simulink model "SF009A_DutyCycThermProtn"  (R2013b)
settings: Solver=FixedStepDiscrete  SolverMode=SingleTasking  StartTime=0.0  StopTime=1  FixedStep=0.1  RelTol=1e-3
values from neighbouring files (symbols this model uses):
  AbsltTThermLimCnt = DataDict.NTC    [SF009A_DutyCycThermProtn_DataDict.m]
  ARCHGLBPRM_100MILLISEC_SEC_F32 = DataDict.Constant    [SF009A_DutyCycThermProtn_DataDict.m]
  CTRLRANDCUTFLT_CNT_U08 = DataDict.Constant    [SF009A_DutyCycThermProtn_DataDict.m]
  CTRLRTFLT_CNT_U08 = DataDict.Constant    [SF009A_DutyCycThermProtn_DataDict.m]
  CUTFLT_CNT_U08 = DataDict.Constant    [SF009A_DutyCycThermProtn_DataDict.m]
  DITHERMLIM_MOTNWTMTR_F32 = DataDict.Constant    [SF009A_DutyCycThermProtn_DataDict.m]
  DutyCycExcddCnt = DataDict.NTC    [SF009A_DutyCycThermProtn_DataDict.m]
  DutyCycThermProtnAbsltCtrlTTblX = DataDict.Calibration    [SF009A_DutyCycThermProtn_DataDict.m]
  DutyCycThermProtnAbsltCtrlTTqTblY = DataDict.Calibration    [SF009A_DutyCycThermProtn_DataDict.m]
  DutyCycThermProtnAbsltCuTTblX = DataDict.Calibration    [SF009A_DutyCycThermProtn_DataDict.m]
  DutyCycThermProtnAbsltCuTTqTblY = DataDict.Calibration    [SF009A_DutyCycThermProtn_DataDict.m]
  DutyCycThermProtnAbsltMotVelBreakPt = DataDict.Calibration    [SF009A_DutyCycThermProtn_DataDict.m]
  DutyCycThermProtnAbsltTTqSlewHiLim = DataDict.Calibration    [SF009A_DutyCycThermProtn_DataDict.m]
  DutyCycThermProtnAbsltTTqSlewLoLim = DataDict.Calibration    [SF009A_DutyCycThermProtn_DataDict.m]
  DutyCycThermProtnCtrlT = DataDict.Calibration    [SF009A_DutyCycThermProtn_DataDict.m]
  DutyCycThermProtnCtrlTSeln = DataDict.Calibration    [SF009A_DutyCycThermProtn_DataDict.m]
  DutyCycThermProtnDutyCycFildThd = DataDict.Calibration    [SF009A_DutyCycThermProtn_DataDict.m]
  DutyCycThermProtnIgnOffCtrlEna = DataDict.Calibration    [SF009A_DutyCycThermProtn_DataDict.m]
  DutyCycThermProtnIgnOffMsgWaitTi = DataDict.Calibration    [SF009A_DutyCycThermProtn_DataDict.m]
  DutyCycThermProtnLstTblValNonStall = DataDict.Calibration    [SF009A_DutyCycThermProtn_DataDict.m]
  DutyCycThermProtnLstTblValStall = DataDict.Calibration    [SF009A_DutyCycThermProtn_DataDict.m]
  DutyCycThermProtnMotPrTSeln = DataDict.Calibration    [SF009A_DutyCycThermProtn_DataDict.m]
  DutyCycThermProtnMplr1NonStallTblY = DataDict.Calibration    [SF009A_DutyCycThermProtn_DataDict.m]
  DutyCycThermProtnMplr1StallTblY = DataDict.Calibration    [SF009A_DutyCycThermProtn_DataDict.m]
  DutyCycThermProtnMplr2NonStallTblY = DataDict.Calibration    [SF009A_DutyCycThermProtn_DataDict.m]
  DutyCycThermProtnMplr2StallTblY = DataDict.Calibration    [SF009A_DutyCycThermProtn_DataDict.m]
  DutyCycThermProtnMplr3NonStallTblY = DataDict.Calibration    [SF009A_DutyCycThermProtn_DataDict.m]
  DutyCycThermProtnMplr3StallTblY = DataDict.Calibration    [SF009A_DutyCycThermProtn_DataDict.m]
  DutyCycThermProtnMplr4NonStallTblY = DataDict.Calibration    [SF009A_DutyCycThermProtn_DataDict.m]
  DutyCycThermProtnMplr4StallTblY = DataDict.Calibration    [SF009A_DutyCycThermProtn_DataDict.m]
  DutyCycThermProtnMplr5NonStallTblY = DataDict.Calibration    [SF009A_DutyCycThermProtn_DataDict.m]
  DutyCycThermProtnMplr5StallTblY = DataDict.Calibration    [SF009A_DutyCycThermProtn_DataDict.m]
  DutyCycThermProtnMplr6NonStallTblY = DataDict.Calibration    [SF009A_DutyCycThermProtn_DataDict.m]
  DutyCycThermProtnMplr6StallTblY = DataDict.Calibration    [SF009A_DutyCycThermProtn_DataDict.m]
  DutyCycThermProtnMplrTblX = DataDict.Calibration    [SF009A_DutyCycThermProtn_DataDict.m]
  DutyCycThermProtnMplrTSeln = DataDict.Calibration    [SF009A_DutyCycThermProtn_DataDict.m]
  DutyCycThermProtnSlowFilTSeln = DataDict.Calibration    [SF009A_DutyCycThermProtn_DataDict.m]
  DutyCycThermProtnThermLimScaFac = DataDict.Calibration    [SF009A_DutyCycThermProtn_DataDict.m]
  DutyCycThermProtnThermLoadLimTblX = DataDict.Calibration    [SF009A_DutyCycThermProtn_DataDict.m]
  DutyCycThermProtnThermLoadLimTblY = DataDict.Calibration    [SF009A_DutyCycThermProtn_DataDict.m]
  DutyCycThermProtnTqCmdSlewDwn = DataDict.Calibration    [SF009A_DutyCycThermProtn_DataDict.m]
  DutyCycThermProtnTqCmdSlewUp = DataDict.Calibration    [SF009A_DutyCycThermProtn_DataDict.m]
  FILVALMIN_ULS_F32 = DataDict.Constant    [SF009A_DutyCycThermProtn_DataDict.m]
  IGNTIOFFTHD_CNT_F32 = DataDict.Constant    [SF009A_DutyCycThermProtn_DataDict.m]
  NODEBSTEP_CNT_U16 = DataDict.Constant    [SF009A_DutyCycThermProtn_DataDict.m]
  ONEPERC_ULS_F32 = DataDict.Constant    [SF009A_DutyCycThermProtn_DataDict.m]
  TAU3_SEC_F32 = DataDict.Constant    [SF009A_DutyCycThermProtn_DataDict.m]
  TAU4_SEC_F32 = DataDict.Constant    [SF009A_DutyCycThermProtn_DataDict.m]
  TAU5_SEC_F32 = DataDict.Constant    [SF009A_DutyCycThermProtn_DataDict.m]
  TAU6_SEC_F32 = DataDict.Constant    [SF009A_DutyCycThermProtn_DataDict.m]
  THERMLOADLIMTBLIDX_ULS_U08 = DataDict.Constant    [SF009A_DutyCycThermProtn_DataDict.m]
undefined symbols (not defined in the file or in its folder): NtcSts1, NvmGetErrSts1
libraries: FixdToFloat x13, Fil x12, NxtrLim x12, simulink x11, NxtrMath x8, FloatToFixd x6, NxtrMax x6, NxtrMin x3, NxtrAbslt x2, NxtrNvM x1
(part 3 of 7)

== system SF009A_DutyCycThermProtn/DutyCycThermProtn/DutyCycThermProtnPer1/ThermalLimitStatus ==
  DutyCycThermProtnDi : Inport
  ThermLim : Inport  Port=2
  Maxout : Inport  Port=3
  CopyRight2 : Subsystem  Description=|  mask(Copyright Information){none=on}
      | Copyright info block.                                               
      |                                                                     
      | Place copyright information at the top of every subsystem in design.
      mask prompts: none "No parameters"
      mask help: Place copyright information at the top of every subsystem in design.
      mask Display:
      | NxtrConf = 'Nexteer Confidential';
      | 
      | sys = bdroot; %handle for the current model ("system")
      | first = get_param(sys,'Created');
      | if(isempty(first))
      |     first = datestr(now,'yyyy');
      | else
      |     first = first(end-3:end);  %year is last four digits
      | end
      | 
      | last = get_param(sys,'LastModifiedDate');
      | if isempty(last)
      |     last = datestr(now,'yyyy');
      | else
      |     last = last(end-3:end);
      | end
      | 
      | if strcmp(first,last)
      |     fprintf('%s -- Copyright %s Nexteer',NxtrConf,first)
      | else
      |     fprintf('%s -- %s%s- %s Nexteer',NxtrConf,char(169),first,last)
      | end
  DutyCycThermProtnDisabled : Subsystem  RequirementInfo={'linktype_rmi_doors' '0000a52a (/E-STEER Core/SubSystem Specifications/Application Functions/SF009A Thermal Duty Cycle Protection)' '#SF009A_267' 'true' 'REQ: SF009A_267' '' } %GIDa_3170260b_8ef3_42fb_9ac5_2884277200d1  TreatAsAtomicUnit=on
  "DutyCycThermProtnEnabled " : Subsystem  RequirementInfo={'linktype_rmi_doors' '0000a52a (/E-STEER Core/SubSystem Specifications/Application Functions/SF009A Thermal Duty Cycle Protection)' '#SF009A_235' 'true' 'REQ: SF009A_235' '' } %GIDa_8d68070d_e413_42c4_a42a_5b349cac34de  TreatAsAtomicUnit=on
  If2 : If  RequirementInfo={'linktype_rmi_doors' '0000a52a (/E-STEER Core/SubSystem Specifications/Application Functions/SF009A Thermal Duty Cycle Protection)' '#SF009A_267' 'true' 'REQ: SF009A_267' '' } %GIDa_d4c54a9c_c30e_44b1_8f16_11f79403e198  IfExpression=u1
  LimStat_f1 : NxtrLim/LimStat_f32  RequirementInfo={'linktype_rmi_doors' '0000a52a (/E-STEER Core/SubSystem Specifications/Application Functions/SF009A Thermal Duty Cycle Protection)' '#SF009A_205' 'true' 'REQ: SF009A_205' '' } %GIDa_2006209c_c7cf_49ec_9d42_30cb8989323e  LoLim=THERMREDNFACLOLIM_ULS_F32  HiLim=THERMREDNFACHILIM_ULS_F32
      settings: AttributesFormatString=Lower Limit: %<LoLim>\nUpper Limit: %<HiLim>
  MaxoutLimiting : Subsystem  RequirementInfo={'linktype_rmi_doors' '0000a52a (/E-STEER Core/SubSystem Specifications/Application Functions/SF009A Thermal Duty Cycle Protection)' '#SF009A_143' 'true' 'REQ: SF009A_143' '' } %GIDa_bba01dfd_191a_49a7_8d73_371fb59628a5  TreatAsAtomicUnit=on
  Merge2 : Merge  RequirementInfo={'linktype_rmi_doors' '0000a52a (/E-STEER Core/SubSystem Specifications/Application Functions/SF009A Thermal Duty Cycle Protection)' '#SF009A_267' 'true' 'REQ: SF009A_267' '' } %GIDa_1305f63a_c873_4a71_994b_19e3fb3df743
  ThermRednFac : Outport
  wires:
  DutyCycThermProtnDi/1 -> MaxoutLimiting/2(DutyCycThermProtnDi), If2/1
  DutyCycThermProtnDisabled/1(ThermRednFac) -> Merge2/1
  If2/1 -> DutyCycThermProtnDisabled/Action
  If2/2 -> "DutyCycThermProtnEnabled "/Action
  LimStat_f1/1 -> ThermRednFac/1
  Merge2/1 -> LimStat_f1/1
  "DutyCycThermProtnEnabled "/1(ThermRednFac) -> Merge2/2
  ThermLim/1 -> "DutyCycThermProtnEnabled "/1(ThermLim)
  Maxout/1 -> MaxoutLimiting/1(Maxout)

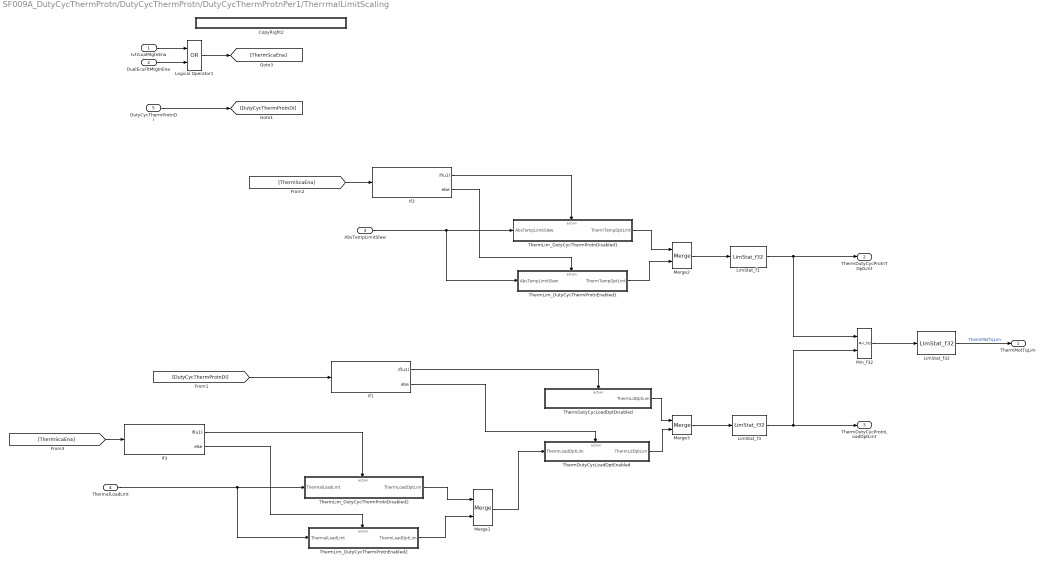
== system SF009A_DutyCycThermProtn/DutyCycThermProtn/DutyCycThermProtnPer1/TherrmalLimitScaling ==
  IvtrLoaMtgtnEna : Inport  RequirementInfo="{'linktype_rmi_doors' '0000a52a (/E-STEER Core/SubSystem Specifications/Application Functions/SF009A Thermal Duty Cycle Protection)' '#SF009A_312' 'true' 'REQ:  SF009A_312' '' } %GIDa_8dc61b0d_ff5c_4fa0_bf26_862789bc8c27"
  DualEcuFltMtgtnEna : Inport  RequirementInfo="{'linktype_rmi_doors' '0000a52a (/E-STEER Core/SubSystem Specifications/Application Functions/SF009A Thermal Duty Cycle Protection)' '#SF009A_312' 'true' 'REQ:  SF009A_312' '' } %GIDa_d897ebab_4d96_4080_9fe6_e7020e9fa09f"  Port=2
  AbsTempLimitSlew : Inport  Port=3
  ThermalLoadLmt : Inport  Port=4
  DutyCycThermProtnDi : Inport  Port=5
  CopyRight2 : Subsystem  Description=|  mask(Copyright Information){none=on}
      | Copyright info block.                                               
      |                                                                     
      | Place copyright information at the top of every subsystem in design.
      mask prompts: none "No parameters"
      mask help: Place copyright information at the top of every subsystem in design.
      mask Display:
      | NxtrConf = 'Nexteer Confidential';
      | 
      | sys = bdroot; %handle for the current model ("system")
      | first = get_param(sys,'Created');
      | first = first(end-3:end);  %year is last four digits
      | 
      | last = get_param(sys,'LastModifiedDate');
      | if isempty(last)
      |     last = datestr(now,'yyyy');
      | else
      |     last = last(end-3:end);
      | end
      | 
      | if strcmp(first,last)
      |     fprintf('%s -- Copyright %s Nexteer',NxtrConf,first)
      | else
      |     fprintf('%s -- %s%s- %s Nexteer',NxtrConf,char(169),first,last)
      | end
  If1 : If  RequirementInfo={} %GIDa_7babfb83_5b52_4390_b634_fda5df83494b  IfExpression=u1
  If2 : If  RequirementInfo={} %GIDa_2cee02fc_25df_4b08_940e_96d0c2f6e22c  IfExpression=u1
  If3 : If  RequirementInfo={} %GIDa_5f0eb570_64b4_4784_95d6_34c2b2a6baa7  IfExpression=u1
  LimStat_f1 : NxtrLim/LimStat_f32  RequirementInfo="{'linktype_rmi_doors' '0000a52a (/E-STEER Core/SubSystem Specifications/Application Functions/SF009A Thermal Duty Cycle Protection)' '#SF009A_309' 'true' 'REQ:  SF009A_309' '' } %GIDa_83c1db68_c9e1_4d9e_932e_8b8cb705e06f"  LoLim=ZERO_MOTNWTMTR_F32  HiLim=SYSGLBPRM_MOTTQCMDHILIM_MOTNWTMTR_F32
      settings: AttributesFormatString=Lower Limit: %<LoLim>\nUpper Limit: %<HiLim>
  LimStat_f3 : NxtrLim/LimStat_f32  RequirementInfo="{'linktype_rmi_doors' '0000a52a (/E-STEER Core/SubSystem Specifications/Application Functions/SF009A Thermal Duty Cycle Protection)' '#SF009A_317' 'true' 'REQ:  SF009A_317' '' } %GIDa_b846f976_f3d0_4532_b6c5_25ce29114272"  LoLim=ZERO_MOTNWTMTR_F32  HiLim=SYSGLBPRM_MOTTQCMDHILIM_MOTNWTMTR_F32
      settings: AttributesFormatString=Lower Limit: %<LoLim>\nUpper Limit: %<HiLim>
  LimStat_f32 : NxtrLim/LimStat_f32  RequirementInfo="{'linktype_rmi_doors' '0000a52a (/E-STEER Core/SubSystem Specifications/Application Functions/SF009A Thermal Duty Cycle Protection)' '#SF009A_318' 'true' 'REQ:  SF009A_318' '' ; 'linktype_rmi_doors' '0000a52a (/E-STEER Core/SubSystem Specifications/Application Functions/SF009A Thermal Duty Cycle Protection)' '#SF009A_319' 'true' 'REQ:  SF009A_319' '' } %GIDa_fa1de0a5_b024_4a72_90f6_53e74d27d671"  LoLim=ZERO_MOTNWTMTR_F32  HiLim=SYSGLBPRM_MOTTQCMDHILIM_MOTNWTMTR_F32
      settings: AttributesFormatString=Lower Limit: %<LoLim>\nUpper Limit: %<HiLim>
  Logical Operator1 : Logic  RequirementInfo="{'linktype_rmi_doors' '0000a52a (/E-STEER Core/SubSystem Specifications/Application Functions/SF009A Thermal Duty Cycle Protection)' '#SF009A_312' 'true' 'REQ:  SF009A_312' '' } %GIDa_a0ab542f_99be_4386_a7f5_35a00b0ad963"  Operator=OR  AllPortsSameDT=off  OutDataTypeStr=boolean
  Merge1 : Merge  RequirementInfo={} %GIDa_d5d1cf90_c902_44f9_82c6_0c36d1509e76
  Merge2 : Merge  RequirementInfo={} %GIDa_d9fd7fe5_0630_493a_b799_686d5074f1b6
  Merge3 : Merge  RequirementInfo={} %GIDa_28a261bc_f2e1_4059_b603_b96f360ef741
  Min_f32 : NxtrMin/Min_f32  SFunctionSpec=single y1 = Min_f32(single u1, single u2)
      settings: AttributesFormatString=%<Name>
  "ThermDutyCycLoadDptDisabled " : Subsystem  RequirementInfo="{'linktype_rmi_doors' '0000a52a (/E-STEER Core/SubSystem Specifications/Application Functions/SF009A Thermal Duty Cycle Protection)' '#SF009A_246' 'true' 'REQ:  SF009A_246' '' } %GIDa_ddc50ac8_1faa_42f8_93ea_c06be95ae3b1"  TreatAsAtomicUnit=on
  ThermDutyCycLoadDptEnabled : Subsystem  RequirementInfo="{'linktype_rmi_doors' '0000a52a (/E-STEER Core/SubSystem Specifications/Application Functions/SF009A Thermal Duty Cycle Protection)' '#SF009A_246' 'true' 'REQ:  SF009A_246' '' } %GIDa_c67cb7cb_e6e1_4854_8d46_a7dea79ca72f"  TreatAsAtomicUnit=on
  ThermLim_DutyCycThermProtnDisabled1 : Subsystem  RequirementInfo="{'linktype_rmi_doors' '0000a52a (/E-STEER Core/SubSystem Specifications/Application Functions/SF009A Thermal Duty Cycle Protection)' '#SF009A_313' 'true' 'REQ:  SF009A_313' '' } %GIDa_2586edea_1805_4e1d_ab84_f723d2ac45af"  TreatAsAtomicUnit=on
  ThermLim_DutyCycThermProtnDisabled2 : Subsystem  RequirementInfo="{'linktype_rmi_doors' '0000a52a (/E-STEER Core/SubSystem Specifications/Application Functions/SF009A Thermal Duty Cycle Protection)' '#SF009A_314' 'true' 'REQ:  SF009A_314' '' } %GIDa_45e1bc34_a818_4763_b74c_1022ecc67c55"  TreatAsAtomicUnit=on
  ThermLim_DutyCycThermProtnEnabled1 : Subsystem  RequirementInfo="{'linktype_rmi_doors' '0000a52a (/E-STEER Core/SubSystem Specifications/Application Functions/SF009A Thermal Duty Cycle Protection)' '#SF009A_313' 'true' 'REQ:  SF009A_313' '' } %GIDa_3bce7b55_05ff_4096_a1dc_b963e5e47b1a"  TreatAsAtomicUnit=on
  ThermLim_DutyCycThermProtnEnabled2 : Subsystem  RequirementInfo="{'linktype_rmi_doors' '0000a52a (/E-STEER Core/SubSystem Specifications/Application Functions/SF009A Thermal Duty Cycle Protection)' '#SF009A_314' 'true' 'REQ:  SF009A_314' '' } %GIDa_331a4316_f4e0_4847_8684_08c003b0afeb"  TreatAsAtomicUnit=on
  ThermMotTqLim : Outport  RequirementInfo="{'linktype_rmi_doors' '0000a52a (/E-STEER Core/SubSystem Specifications/Application Functions/SF009A Thermal Duty Cycle Protection)' '#SF009A_318' 'true' 'REQ:  SF009A_318' '' ; 'linktype_rmi_doors' '0000a52a (/E-STEER Core/SubSystem Specifications/Application Functions/SF009A Thermal Duty Cycle Protection)' '#SF009A_319' 'true' 'REQ:  SF009A_319' '' } %GIDa_a2d08e3e_eec7_4b12_a4b0_81f4b84f2415"
  ThermDutyCycProtnTDptLmt : Outport  RequirementInfo="{'linktype_rmi_doors' '0000a52a (/E-STEER Core/SubSystem Specifications/Application Functions/SF009A Thermal Duty Cycle Protection)' '#SF009A_309' 'true' 'REQ:  SF009A_309' '' } %GIDa_17b4566a_b19b_4e3d_9f2a_5a599306e544"  Port=2
  ThermDutyCycProtnLoadDptLmt : Outport  RequirementInfo="{'linktype_rmi_doors' '0000a52a (/E-STEER Core/SubSystem Specifications/Application Functions/SF009A Thermal Duty Cycle Protection)' '#SF009A_317' 'true' 'REQ:  SF009A_317' '' } %GIDa_b461d353_80d8_421a_910a_1fa039d560eb"  Port=3
  wires:
  LimStat_f32/1 -> ThermMotTqLim/1  "ThermMotTqLim"
  If1/1 -> "ThermDutyCycLoadDptDisabled "/Action
  If1/2 -> ThermDutyCycLoadDptEnabled/Action
  DutyCycThermProtnDi/1 -> [DutyCycThermProtnDi]
  "ThermDutyCycLoadDptDisabled "/1(ThermLdDptLim) -> Merge3/1
  ThermDutyCycLoadDptEnabled/1(ThermLdDptLim) -> Merge3/2
  Merge3/1 -> LimStat_f3/1
  LimStat_f3/1 -> Min_f32/2, ThermDutyCycProtnLoadDptLmt/1
  [DutyCycThermProtnDi] -> If1/1
  IvtrLoaMtgtnEna/1 -> Logical Operator1/1
  DualEcuFltMtgtnEna/1 -> Logical Operator1/2
  Logical Operator1/1 -> [ThermScaEna]
  [ThermScaEna] -> If2/1
  If2/1 -> ThermLim_DutyCycThermProtnDisabled1/Action
  AbsTempLimitSlew/1 -> ThermLim_DutyCycThermProtnEnabled1/1(AbsTempLimitSlew), ThermLim_DutyCycThermProtnDisabled1/1(AbsTempLimitSlew)
  If2/2 -> ThermLim_DutyCycThermProtnEnabled1/Action
  ThermLim_DutyCycThermProtnDisabled1/1(ThermTempDptLmt) -> Merge2/1
  ThermLim_DutyCycThermProtnEnabled1/1(ThermTempDptLmt) -> Merge2/2
  Merge2/1 -> LimStat_f1/1
  LimStat_f1/1 -> Min_f32/1, ThermDutyCycProtnTDptLmt/1
  [ThermScaEna] -> If3/1
  If3/1 -> ThermLim_DutyCycThermProtnDisabled2/Action
  ThermalLoadLmt/1 -> ThermLim_DutyCycThermProtnEnabled2/1(ThermalLoadLmt), ThermLim_DutyCycThermProtnDisabled2/1(ThermalLoadLmt)
  If3/2 -> ThermLim_DutyCycThermProtnEnabled2/Action
  ThermLim_DutyCycThermProtnDisabled2/1(ThermLoadDptLim) -> Merge1/1
  ThermLim_DutyCycThermProtnEnabled2/1(ThermLoadDptLim) -> Merge1/2
  Merge1/1 -> ThermDutyCycLoadDptEnabled/1(ThermLoadDptLim)
  Min_f32/1 -> LimStat_f32/1

== system SF009A_DutyCycThermProtn/DutyCycThermProtn/DutyCycThermProtnInit1/FilStVal_SetRamBlockStatus/CopyRight2 ==

== system SF009A_DutyCycThermProtn/DutyCycThermProtn/DutyCycThermProtnInit1/NVM_NOK/CopyRight2 ==

== system SF009A_DutyCycThermProtn/DutyCycThermProtn/DutyCycThermProtnInit1/NVM_Ok/CopyRight2 ==

== system SF009A_DutyCycThermProtn/DutyCycThermProtn/DutyCycThermProtnInit1/PowerOnTasks/CopyRight2 ==

== system SF009A_DutyCycThermProtn/DutyCycThermProtn/DutyCycThermProtnInit1/PowerOnTasks/DefaultIgnOffTime ==
  Action Port : ActionPort  ActionType=else
  CopyRight2 : Subsystem  Description=|  mask(Copyright Information){none=on}
      | Copyright info block.                                               
      |                                                                     
      | Place copyright information at the top of every subsystem in design.
      mask prompts: none "No parameters"
      mask help: Place copyright information at the top of every subsystem in design.
      mask Display:
      | NxtrConf = 'Nexteer Confidential';
      | 
      | sys = bdroot; %handle for the current model ("system")
      | first = get_param(sys,'Created');
      | first = first(end-3:end);  %year is last four digits
      | 
      | last = get_param(sys,'LastModifiedDate');
      | if isempty(last)
      |     last = datestr(now,'yyyy');
      | else
      |     last = last(end-3:end);
      | end
      | 
      | if strcmp(first,last)
      |     fprintf('%s -- Copyright %s Nexteer',NxtrConf,first)
      | else
      |     fprintf('%s -- %s%s- %s Nexteer',NxtrConf,char(169),first,last)
      | end
  DefIgnOffTime1 : Constant  RequirementInfo={'linktype_rmi_doors' '0000a52a (/E-STEER Core/SubSystem Specifications/Application Functions/SF009A Thermal Duty Cycle Protection)' '#SF009A_285' 'true' 'REQ: SF009A_285' '' } %GIDa_1c1a8355_68c4_4a16_a698_2c7b860aa81f  Value=FILVALMIN_ULS_F32
  FiltSV3 : Outport  RequirementInfo={'linktype_rmi_doors' '0000a52a (/E-STEER Core/SubSystem Specifications/Application Functions/SF009A Thermal Duty Cycle Protection)' '#SF009A_285' 'true' 'REQ: SF009A_285' '' } %GIDa_f53f9a1c_8faf_4833_a80c_e2891c436a6f
  FiltSV4 : Outport  RequirementInfo={'linktype_rmi_doors' '0000a52a (/E-STEER Core/SubSystem Specifications/Application Functions/SF009A Thermal Duty Cycle Protection)' '#SF009A_285' 'true' 'REQ: SF009A_285' '' } %GIDa_7573da05_c607_444c_bff7_05b9be356769  Port=2
  FiltSV5 : Outport  RequirementInfo={'linktype_rmi_doors' '0000a52a (/E-STEER Core/SubSystem Specifications/Application Functions/SF009A Thermal Duty Cycle Protection)' '#SF009A_285' 'true' 'REQ: SF009A_285' '' } %GIDa_0a22d052_a9b5_4254_83f4_8f154e55c7ba  Port=3
  FiltSV6 : Outport  RequirementInfo={'linktype_rmi_doors' '0000a52a (/E-STEER Core/SubSystem Specifications/Application Functions/SF009A Thermal Duty Cycle Protection)' '#SF009A_285' 'true' 'REQ: SF009A_285' '' } %GIDa_7f0b1c6f_6523_47e0_8553_42c05ca6b0db  Port=4
  wires:
  DefIgnOffTime1/1 -> FiltSV3/1, FiltSV4/1, FiltSV6/1, FiltSV5/1

== system SF009A_DutyCycThermProtn/DutyCycThermProtn/DutyCycThermProtnInit1/PowerOnTasks/InputIgnOffTime ==
  note: RANGE CHECK, ENSURE VALUE IS BELOW A CONSTANT (10000)
  IgnTiOff : Inport
  Action Port : ActionPort  ActionType=then
  CopyRight2 : Subsystem  Description=|  mask(Copyright Information){none=on}
      | Copyright info block.                                               
      |                                                                     
      | Place copyright information at the top of every subsystem in design.
      mask prompts: none "No parameters"
      mask help: Place copyright information at the top of every subsystem in design.
      mask Display:
      | NxtrConf = 'Nexteer Confidential';
      | 
      | sys = bdroot; %handle for the current model ("system")
      | first = get_param(sys,'Created');
      | first = first(end-3:end);  %year is last four digits
      | 
      | last = get_param(sys,'LastModifiedDate');
      | if isempty(last)
      |     last = datestr(now,'yyyy');
      | else
      |     last = last(end-3:end);
      | end
      | 
      | if strcmp(first,last)
      |     fprintf('%s -- Copyright %s Nexteer',NxtrConf,first)
      | else
      |     fprintf('%s -- %s%s- %s Nexteer',NxtrConf,char(169),first,last)
      | end
  Data Store Read : DataStoreRead  DataStoreName=FilStVal  DataStoreElements=FilStVal.Fil3StVal
  Data Store Read1 : DataStoreRead  DataStoreName=FilStVal  DataStoreElements=FilStVal.Fil4StVal
  Data Store Read2 : DataStoreRead  DataStoreName=FilStVal  DataStoreElements=FilStVal.Fil5StVal
  Data Store Read3 : DataStoreRead  DataStoreName=FilStVal  DataStoreElements=FilStVal.Fil6StVal
  Filt3ExpDecay : Subsystem  RequirementInfo={} %GIDa_9f9f3f65_c145_44e4_82e5_fd713760ae68
  Filt4ExpDecay : Subsystem  RequirementInfo={} %GIDa_626963e8_8ecf_441f_b1c9_4240579d77f9
  Filt5ExpDecay : Subsystem  RequirementInfo={} %GIDa_9364c89b_18fa_4473_8499_21374c540da9
  Filt6ExpDecay : Subsystem  RequirementInfo={} %GIDa_8e6049b9_bd81_40a5_96f3_6037c184dcb3
  FiltSV3 : Outport
  FiltSV4 : Outport  Port=2
  FiltSV5 : Outport  Port=3
  FiltSV6 : Outport  Port=4
  wires:
  Filt3ExpDecay/1(FiltSV) -> FiltSV3/1
  Data Store Read/1 -> Filt3ExpDecay/2(FiltSVOrg)
  Filt4ExpDecay/1(FiltSV) -> FiltSV4/1
  Filt5ExpDecay/1(FiltSV) -> FiltSV5/1
  Data Store Read2/1 -> Filt5ExpDecay/2(FiltSVOrg)
  Filt6ExpDecay/1(FiltSV) -> FiltSV6/1
  Data Store Read3/1 -> Filt6ExpDecay/2(FiltSVOrg)
  Data Store Read1/1 -> Filt4ExpDecay/2(FiltSVOrg)
  IgnTiOff/1 -> Filt3ExpDecay/1(IgnTimeOffSel), Filt4ExpDecay/1(IgnTimeOffSel), Filt6ExpDecay/1(IgnTimeOffSel), Filt5ExpDecay/1(IgnTimeOffSel)

== system SF009A_DutyCycThermProtn/DutyCycThermProtn/DutyCycThermProtnInit1/SetInitialValueOfAbsTempLimitSlew/Copyright1 ==

== system SF009A_DutyCycThermProtn/DutyCycThermProtn/DutyCycThermProtnInit1/SetInitialValueOfLstTblValRateLimrStVari/Copyright1 ==

== system SF009A_DutyCycThermProtn/DutyCycThermProtn/DutyCycThermProtnPer1/FiltSVReinit/CopyRight2 ==

== system SF009A_DutyCycThermProtn/DutyCycThermProtn/DutyCycThermProtnPer1/FiltSVReinit/VehTiVldDisabled ==
  Action Port : ActionPort  ActionType=else
  CopyRight2 : Subsystem  Description=|  mask(Copyright Information){none=on}
      | Copyright info block.                                               
      |                                                                     
      | Place copyright information at the top of every subsystem in design.
      mask prompts: none "No parameters"
      mask help: Place copyright information at the top of every subsystem in design.
      mask Display:
      | NxtrConf = 'Nexteer Confidential';
      | 
      | sys = bdroot; %handle for the current model ("system")
      | first = get_param(sys,'Created');
      | first = first(end-3:end);  %year is last four digits
      | 
      | last = get_param(sys,'LastModifiedDate');
      | if isempty(last)
      |     last = datestr(now,'yyyy');
      | else
      |     last = last(end-3:end);
      | end
      | 
      | if strcmp(first,last)
      |     fprintf('%s -- Copyright %s Nexteer',NxtrConf,first)
      | else
      |     fprintf('%s -- %s%s- %s Nexteer',NxtrConf,char(169),first,last)
      | end
  DefIgnOffTime1 : Constant  RequirementInfo={'linktype_rmi_doors' '0000a52a (/E-STEER Core/SubSystem Specifications/Application Functions/SF009A Thermal Duty Cycle Protection)' '#SF009A_285' 'true' 'REQ: SF009A_285' '' } %GIDa_ff571b1a_1782_4f5b_8061_ceec6519b3d1  Value=FILVALMIN_ULS_F32
  FiltSV3 : Outport  RequirementInfo={'linktype_rmi_doors' '0000a52a (/E-STEER Core/SubSystem Specifications/Application Functions/SF009A Thermal Duty Cycle Protection)' '#SF009A_285' 'true' 'REQ: SF009A_285' '' } %GIDa_7dd21f81_ccc7_49b6_9939_90cfad62de91
  FiltSV4 : Outport  RequirementInfo={'linktype_rmi_doors' '0000a52a (/E-STEER Core/SubSystem Specifications/Application Functions/SF009A Thermal Duty Cycle Protection)' '#SF009A_285' 'true' 'REQ: SF009A_285' '' } %GIDa_9e3d7e87_4137_4c20_943f_e98c68156777  Port=2
  FiltSV5 : Outport  RequirementInfo={'linktype_rmi_doors' '0000a52a (/E-STEER Core/SubSystem Specifications/Application Functions/SF009A Thermal Duty Cycle Protection)' '#SF009A_285' 'true' 'REQ: SF009A_285' '' } %GIDa_7d2d2855_4602_487a_979b_6bffe0216b93  Port=3
  FiltSV6 : Outport  RequirementInfo={'linktype_rmi_doors' '0000a52a (/E-STEER Core/SubSystem Specifications/Application Functions/SF009A Thermal Duty Cycle Protection)' '#SF009A_285' 'true' 'REQ: SF009A_285' '' } %GIDa_d4f64410_e786_41b0_841d_daea9815ca41  Port=4
  wires:
  DefIgnOffTime1/1 -> FiltSV3/1, FiltSV4/1, FiltSV6/1, FiltSV5/1

== system SF009A_DutyCycThermProtn/DutyCycThermProtn/DutyCycThermProtnPer1/FiltSVReinit/VehTiVldEnabled ==
  IgnTiOff : Inport
  Action Port : ActionPort  ActionType=then
  CopyRight2 : Subsystem  Description=|  mask(Copyright Information){none=on}
      | Copyright info block.                                               
      |                                                                     
      | Place copyright information at the top of every subsystem in design.
      mask prompts: none "No parameters"
      mask help: Place copyright information at the top of every subsystem in design.
      mask Display:
      | NxtrConf = 'Nexteer Confidential';
      | 
      | sys = bdroot; %handle for the current model ("system")
      | first = get_param(sys,'Created');
      | first = first(end-3:end);  %year is last four digits
      | 
      | last = get_param(sys,'LastModifiedDate');
      | if isempty(last)
      |     last = datestr(now,'yyyy');
      | else
      |     last = last(end-3:end);
      | end
      | 
      | if strcmp(first,last)
      |     fprintf('%s -- Copyright %s Nexteer',NxtrConf,first)
      | else
      |     fprintf('%s -- %s%s- %s Nexteer',NxtrConf,char(169),first,last)
      | end
  Data Store Read : DataStoreRead  DataStoreName=Fil3ValPwrUp
  Data Store Read1 : DataStoreRead  DataStoreName=Fil4ValPwrUp
  Data Store Read2 : DataStoreRead  DataStoreName=Fil5ValPwrUp
  Data Store Read3 : DataStoreRead  DataStoreName=Fil6ValPwrUp
  Filt3ExpDecay : Subsystem
  Filt4ExpDecay : Subsystem
  Filt5ExpDecay : Subsystem
  Filt6ExpDecay : Subsystem
  FiltSV3 : Outport
  FiltSV4 : Outport  Port=2
  FiltSV5 : Outport  Port=3
  FiltSV6 : Outport  Port=4
  wires:
  IgnTiOff/1 -> Filt6ExpDecay/1(IgnTimeOffSel), Filt5ExpDecay/1(IgnTimeOffSel), Filt4ExpDecay/1(IgnTimeOffSel), Filt3ExpDecay/1(IgnTimeOffSel)
  Data Store Read3/1 -> Filt6ExpDecay/2(FiltSVOrg)
  Filt6ExpDecay/1(FiltSV) -> FiltSV6/1
  Data Store Read2/1 -> Filt5ExpDecay/2(FiltSVOrg)
  Filt5ExpDecay/1(FiltSV) -> FiltSV5/1
  Data Store Read1/1 -> Filt4ExpDecay/2(FiltSVOrg)
  Filt4ExpDecay/1(FiltSV) -> FiltSV4/1
  Data Store Read/1 -> Filt3ExpDecay/2(FiltSVOrg)
  Filt3ExpDecay/1(FiltSV) -> FiltSV3/1

== system SF009A_DutyCycThermProtn/DutyCycThermProtn/DutyCycThermProtnPer1/LoadLimiting/CopyRight2 ==

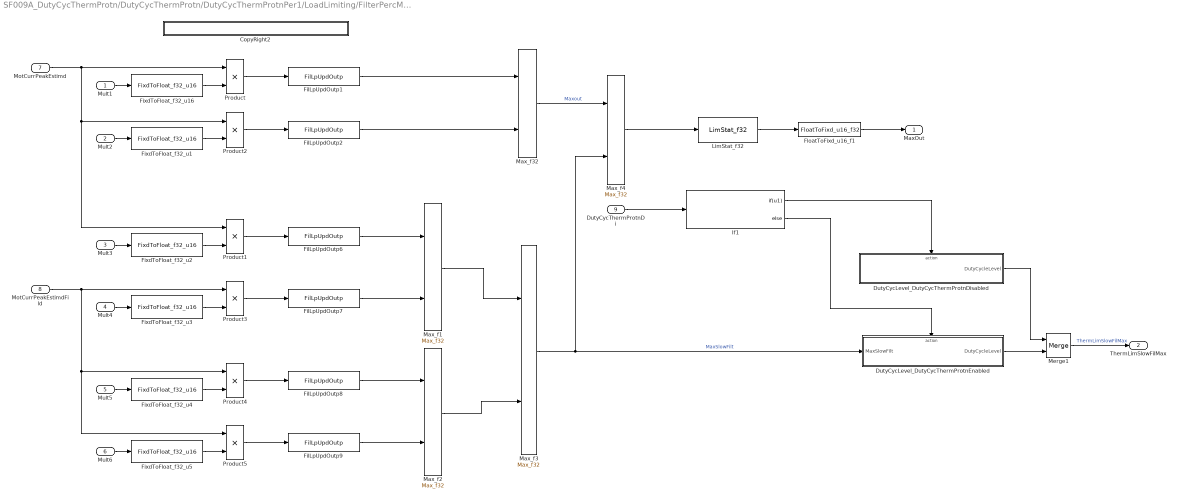
== system SF009A_DutyCycThermProtn/DutyCycThermProtn/DutyCycThermProtnPer1/LoadLimiting/FilterPercMax ==
  Mult1 : Inport
  Mult2 : Inport  Port=2
  Mult3 : Inport  Port=3
  Mult4 : Inport  Port=4
  Mult5 : Inport  Port=5
  Mult6 : Inport  Port=6
  MotCurrPeakEstimd : Inport  Port=7
  MotCurrPeakEstimdFild : Inport  Port=8
  DutyCycThermProtnDi : Inport  Port=9
  CopyRight2 : Subsystem  Description=|  mask(Copyright Information){none=on}
      | Copyright info block.                                               
      |                                                                     
      | Place copyright information at the top of every subsystem in design.
      mask prompts: none "No parameters"
      mask help: Place copyright information at the top of every subsystem in design.
      mask Display:
      | NxtrConf = 'Nexteer Confidential';
      | 
      | sys = bdroot; %handle for the current model ("system")
      | first = get_param(sys,'Created');
      | first = first(end-3:end);  %year is last four digits
      | 
      | last = get_param(sys,'LastModifiedDate');
      | if isempty(last)
      |     last = datestr(now,'yyyy');
      | else
      |     last = last(end-3:end);
      | end
      | 
      | if strcmp(first,last)
      |     fprintf('%s -- Copyright %s Nexteer',NxtrConf,first)
      | else
      |     fprintf('%s -- %s%s- %s Nexteer',NxtrConf,char(169),first,last)
      | end
  DutyCycLevel_DutyCycThermProtnDisabled : Subsystem  RequirementInfo={'linktype_rmi_doors' '0000a52a (/E-STEER Core/SubSystem Specifications/Application Functions/SF009A Thermal Duty Cycle Protection)' '#SF009A_168' 'true' 'REQ: SF009A_168' '' } %GIDa_71363024_cb12_46dd_971c_3c161e9d529d  TreatAsAtomicUnit=on
  DutyCycLevel_DutyCycThermProtnEnabled : Subsystem  RequirementInfo={'linktype_rmi_doors' '0000a52a (/E-STEER Core/SubSystem Specifications/Application Functions/SF009A Thermal Duty Cycle Protection)' '#SF009A_168' 'true' 'REQ: SF009A_168' '' } %GIDa_1862e0cc_48c0_4a64_b3aa_9ef2fa11f229  TreatAsAtomicUnit=on
  FilLpUpdOutp1 : Fil/FilLpUpdOutp  RequirementInfo={'linktype_rmi_doors' '0000a52a (/E-STEER Core/SubSystem Specifications/Application Functions/SF009A Thermal Duty Cycle Protection)' '#SF009A_117' 'true' 'REQ: SF009A_117' '' } %GIDa_36d69916_80a2_4684_8052_fd4d54618007  StVar=Fil1ValStVari
      settings: AttributesFormatString=StVar: %<StVar>
  FilLpUpdOutp2 : Fil/FilLpUpdOutp  RequirementInfo={'linktype_rmi_doors' '0000a52a (/E-STEER Core/SubSystem Specifications/Application Functions/SF009A Thermal Duty Cycle Protection)' '#SF009A_117' 'true' 'REQ: SF009A_117' '' } %GIDa_9334f7f9_570f_473a_a841_bd6f3c21f9df  StVar=Fil2ValStVari
      settings: AttributesFormatString=StVar: %<StVar>
  FilLpUpdOutp6 : Fil/FilLpUpdOutp  RequirementInfo={'linktype_rmi_doors' '0000a52a (/E-STEER Core/SubSystem Specifications/Application Functions/SF009A Thermal Duty Cycle Protection)' '#SF009A_117' 'true' 'REQ: SF009A_117' '' } %GIDa_8cd640f7_4fe0_46fd_98bb_13b2eab9fb91  StVar=Fild3Val
      settings: AttributesFormatString=StVar: %<StVar>
  FilLpUpdOutp7 : Fil/FilLpUpdOutp  RequirementInfo={'linktype_rmi_doors' '0000a52a (/E-STEER Core/SubSystem Specifications/Application Functions/SF009A Thermal Duty Cycle Protection)' '#SF009A_117' 'true' 'REQ: SF009A_117' '' } %GIDa_84154e02_2e1c_41ac_9811_25a1fbb85ef4  StVar=Fild4Val
      settings: AttributesFormatString=StVar: %<StVar>
  FilLpUpdOutp8 : Fil/FilLpUpdOutp  RequirementInfo={'linktype_rmi_doors' '0000a52a (/E-STEER Core/SubSystem Specifications/Application Functions/SF009A Thermal Duty Cycle Protection)' '#SF009A_117' 'true' 'REQ: SF009A_117' '' } %GIDa_4a9913a0_954a_4382_b1cf_522ede446f9f  StVar=Fild5Val
      settings: AttributesFormatString=StVar: %<StVar>
  FilLpUpdOutp9 : Fil/FilLpUpdOutp  RequirementInfo={'linktype_rmi_doors' '0000a52a (/E-STEER Core/SubSystem Specifications/Application Functions/SF009A Thermal Duty Cycle Protection)' '#SF009A_117' 'true' 'REQ: SF009A_117' '' } %GIDa_c55f5e10_5865_48ee_8ffc_2f75da5ed5de  StVar=Fild6Val
      settings: AttributesFormatString=StVar: %<StVar>
  FixdToFloat_f32_u{1..5,16} (6 alike) : FixdToFloat/FixdToFloat_f32_u16  Param1=13
  FloatToFixd_u16_f1 : FloatToFixd/FloatToFixd_u16_f32  Param1=0
  If1 : If  RequirementInfo={'linktype_rmi_doors' '0000a52a (/E-STEER Core/SubSystem Specifications/Application Functions/SF009A Thermal Duty Cycle Protection)' '#SF009A_168' 'true' 'REQ: SF009A_168' '' } %GIDa_157cb9dd_8c28_4ea7_a2f6_9f40ccd5ede0  IfExpression=u1
  LimStat_f32 : NxtrLim/LimStat_f32  LoLim=single(0)  HiLim=FILOUTPLIM_ULS_F32
      settings: AttributesFormatString=Lower Limit: %<LoLim>\nUpper Limit: %<HiLim>
  Max_f1 : NxtrMax/Max_f32  RequirementInfo={'linktype_rmi_doors' '0000a52a (/E-STEER Core/SubSystem Specifications/Application Functions/SF009A Thermal Duty Cycle Protection)' '#SF009A_164' 'true' 'REQ: SF009A_164' '' ; 'linktype_rmi_doors' '0000a52a (/E-STEER Core/SubSystem Specifications/Application Functions/SF009A Thermal Duty Cycle Protection)' '#SF009A_167' 'true' 'REQ: SF009A_167' '' } %GIDa_ca8925de_f515_4e09_b430_d40efee02347  SFunctionSpec=single y1 = Max_f32(single u1, single u2)
  Max_f2 : NxtrMax/Max_f32  RequirementInfo={'linktype_rmi_doors' '0000a52a (/E-STEER Core/SubSystem Specifications/Application Functions/SF009A Thermal Duty Cycle Protection)' '#SF009A_164' 'true' 'REQ: SF009A_164' '' ; 'linktype_rmi_doors' '0000a52a (/E-STEER Core/SubSystem Specifications/Application Functions/SF009A Thermal Duty Cycle Protection)' '#SF009A_167' 'true' 'REQ: SF009A_167' '' } %GIDa_b559abac_2e26_4623_b247_6a9c382bd671  SFunctionSpec=single y1 = Max_f32(single u1, single u2)
  Max_f3 : NxtrMax/Max_f32  RequirementInfo={'linktype_rmi_doors' '0000a52a (/E-STEER Core/SubSystem Specifications/Application Functions/SF009A Thermal Duty Cycle Protection)' '#SF009A_164' 'true' 'REQ: SF009A_164' '' ; 'linktype_rmi_doors' '0000a52a (/E-STEER Core/SubSystem Specifications/Application Functions/SF009A Thermal Duty Cycle Protection)' '#SF009A_167' 'true' 'REQ: SF009A_167' '' } %GIDa_092cd743_3616_45d9_acc8_4304d3de2e74  SFunctionSpec=single y1 = Max_f32(single u1, single u2)
  Max_f32 : NxtrMax/Max_f32  RequirementInfo={'linktype_rmi_doors' '0000a52a (/E-STEER Core/SubSystem Specifications/Application Functions/SF009A Thermal Duty Cycle Protection)' '#SF009A_164' 'true' 'REQ: SF009A_164' '' } %GIDa_d19587f6_c498_4d64_88b0_72feb27fc8ad  SFunctionSpec=single y1 = Max_f32(single u1, single u2)
  Max_f4 : NxtrMax/Max_f32  RequirementInfo={'linktype_rmi_doors' '0000a52a (/E-STEER Core/SubSystem Specifications/Application Functions/SF009A Thermal Duty Cycle Protection)' '#SF009A_164' 'true' 'REQ: SF009A_164' '' } %GIDa_8231735f_1900_427b_8d69_95be75866dae  SFunctionSpec=single y1 = Max_f32(single u1, single u2)
  Merge1 : Merge  RequirementInfo={'linktype_rmi_doors' '0000a52a (/E-STEER Core/SubSystem Specifications/Application Functions/SF009A Thermal Duty Cycle Protection)' '#SF009A_168' 'true' 'REQ: SF009A_168' '' } %GIDa_7470e7ba_5e3d_450c_abd9_7a59ae4fb17e
  Product{,1..5} (6 alike) : Product  RndMeth=Zero
  MaxOut : Outport
  ThermLimSlowFilMax : Outport  RequirementInfo={'linktype_rmi_doors' '0000a52a (/E-STEER Core/SubSystem Specifications/Application Functions/SF009A Thermal Duty Cycle Protection)' '#SF009A_257' 'true' 'REQ: SF009A_257' '' } %GIDa_486bc804_3010_4761_b204_bb6960c359d5  Port=2
  wires:
  FilLpUpdOutp6/1 -> Max_f1/1
  Max_f1/1 -> Max_f3/1
  LimStat_f32/1 -> FloatToFixd_u16_f1/1
  FilLpUpdOutp7/1 -> Max_f1/2
  FilLpUpdOutp8/1 -> Max_f2/1
  FilLpUpdOutp9/1 -> Max_f2/2
  Merge1/1 -> ThermLimSlowFilMax/1  "ThermLimSlowFilMax"
  MotCurrPeakEstimd/1 -> Product2/1, Product1/1, Product/1
  Mult1/1 -> FixdToFloat_f32_u16/1
  Mult3/1 -> FixdToFloat_f32_u2/1
  Mult2/1 -> FixdToFloat_f32_u1/1
  Product/1 -> FilLpUpdOutp1/1
  MotCurrPeakEstimdFild/1 -> Product3/1, Product5/1, Product4/1
  Mult4/1 -> FixdToFloat_f32_u3/1
  Mult5/1 -> FixdToFloat_f32_u4/1
  Mult6/1 -> FixdToFloat_f32_u5/1
  Product2/1 -> FilLpUpdOutp2/1
  Product1/1 -> FilLpUpdOutp6/1
  Product3/1 -> FilLpUpdOutp7/1
  Product4/1 -> FilLpUpdOutp8/1
  Product5/1 -> FilLpUpdOutp9/1
  FilLpUpdOutp1/1 -> Max_f32/1
  FilLpUpdOutp2/1 -> Max_f32/2
  DutyCycThermProtnDi/1 -> If1/1
  DutyCycLevel_DutyCycThermProtnDisabled/1(DutyCycleLevel) -> Merge1/1
  DutyCycLevel_DutyCycThermProtnEnabled/1(DutyCycleLevel) -> Merge1/2
  Max_f4/1 -> LimStat_f32/1
  If1/1 -> DutyCycLevel_DutyCycThermProtnDisabled/Action
  If1/2 -> DutyCycLevel_DutyCycThermProtnEnabled/Action
  Max_f2/1 -> Max_f3/2
  Max_f3/1 -> DutyCycLevel_DutyCycThermProtnEnabled/1(MaxSlowFilt), Max_f4/2  "MaxSlowFilt"
  Max_f32/1 -> Max_f4/1  "Maxout"
  FixdToFloat_f32_u16/1 -> Product/2
  FixdToFloat_f32_u1/1 -> Product2/2
  FixdToFloat_f32_u2/1 -> Product1/2
  FixdToFloat_f32_u3/1 -> Product3/2
  FixdToFloat_f32_u4/1 -> Product4/2
  FixdToFloat_f32_u5/1 -> Product5/2
  FloatToFixd_u16_f1/1 -> MaxOut/1

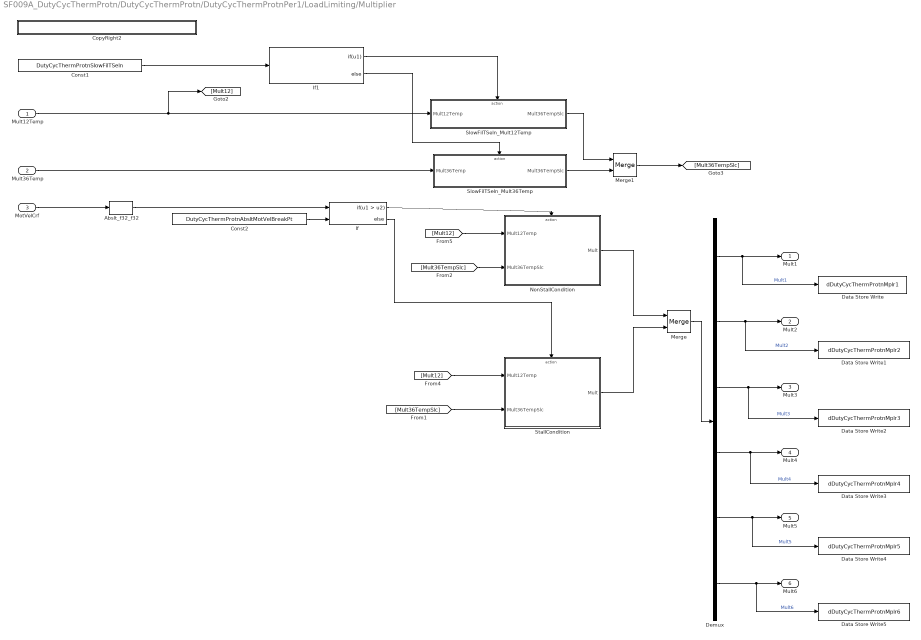
== system SF009A_DutyCycThermProtn/DutyCycThermProtn/DutyCycThermProtnPer1/LoadLimiting/Multiplier ==
  Mult12Temp : Inport
  Mult36Temp : Inport  Port=2
  MotVelCrf : Inport  Port=3
  Abslt_f32_f32 : NxtrAbslt/Abslt_f32_f32  SFunctionSpec=single y1 = Abslt_f32_f32(single u1)
      settings: AttributesFormatString=%<Name>
  Const1 : Constant  RequirementInfo={'linktype_rmi_doors' '0000a52a (/E-STEER Core/SubSystem Specifications/Application Functions/SF009A Thermal Duty Cycle Protection)' '#SF009A_151' 'true' 'REQ: SF009A_151' '' } %GIDa_87016093_dca7_4680_b392_3511aa636729  Value=DutyCycThermProtnSlowFilTSeln
  Const2 : Constant  RequirementInfo={'linktype_rmi_doors' '0000a52a (/E-STEER Core/SubSystem Specifications/Application Functions/SF009A Thermal Duty Cycle Protection)' '#SF009A_217' 'true' 'REQ: SF009A_217' '' } %GIDa_e07e7f93_d6c7_47ef_bf2e_19c09e4ab3f5  Value=DutyCycThermProtnAbsltMotVelBreakPt
  CopyRight2 : Subsystem  Description=|  mask(Copyright Information){none=on}
      | Copyright info block.                                               
      |                                                                     
      | Place copyright information at the top of every subsystem in design.
      mask prompts: none "No parameters"
      mask help: Place copyright information at the top of every subsystem in design.
      mask Display:
      | NxtrConf = 'Nexteer Confidential';
      | 
      | sys = bdroot; %handle for the current model ("system")
      | first = get_param(sys,'Created');
      | first = first(end-3:end);  %year is last four digits
      | 
      | last = get_param(sys,'LastModifiedDate');
      | if isempty(last)
      |     last = datestr(now,'yyyy');
      | else
      |     last = last(end-3:end);
      | end
      | 
      | if strcmp(first,last)
      |     fprintf('%s -- Copyright %s Nexteer',NxtrConf,first)
      | else
      |     fprintf('%s -- %s%s- %s Nexteer',NxtrConf,char(169),first,last)
      | end
  Data Store Write : DataStoreWrite  DataStoreName=dDutyCycThermProtnMplr1
  Data Store Write1 : DataStoreWrite  DataStoreName=dDutyCycThermProtnMplr2
  Data Store Write2 : DataStoreWrite  DataStoreName=dDutyCycThermProtnMplr3
  Data Store Write3 : DataStoreWrite  DataStoreName=dDutyCycThermProtnMplr4
  Data Store Write4 : DataStoreWrite  DataStoreName=dDutyCycThermProtnMplr5
  Data Store Write5 : DataStoreWrite  DataStoreName=dDutyCycThermProtnMplr6
  Demux : Demux  Outputs=6
  If : If  RequirementInfo={'linktype_rmi_doors' '0000a52a (/E-STEER Core/SubSystem Specifications/Application Functions/SF009A Thermal Duty Cycle Protection)' '#SF009A_116' 'true' 'REQ: SF009A_116' '' } %GIDa_d0360e02_97ce_48cf_8672_eb1c09016105  NumInputs=2  IfExpression=u1 > u2
  If1 : If  RequirementInfo={'linktype_rmi_doors' '0000a52a (/E-STEER Core/SubSystem Specifications/Application Functions/SF009A Thermal Duty Cycle Protection)' '#SF009A_151' 'true' 'REQ: SF009A_151' '' } %GIDa_2f381bbc_50d4_414d_93a6_c1ebc2063f26  IfExpression=u1
  Merge : Merge  RequirementInfo={'linktype_rmi_doors' '0000a52a (/E-STEER Core/SubSystem Specifications/Application Functions/SF009A Thermal Duty Cycle Protection)' '#SF009A_116' 'true' 'REQ: SF009A_116' '' } %GIDa_424897de_be3d_4953_97de_501b9efc0782
  Merge1 : Merge  RequirementInfo={'linktype_rmi_doors' '0000a52a (/E-STEER Core/SubSystem Specifications/Application Functions/SF009A Thermal Duty Cycle Protection)' '#SF009A_151' 'true' 'REQ: SF009A_151' '' } %GIDa_8d80e534_1858_41f5_a507_1f5b1fd28779
  NonStallCondition : Subsystem  RequirementInfo={'linktype_rmi_doors' '0000a52a (/E-STEER Core/SubSystem Specifications/Application Functions/SF009A Thermal Duty Cycle Protection)' '#SF009A_116' 'true' 'REQ: SF009A_116' '' } %GIDa_c13999ff_915f_4750_b6af_90471e97e0b1  TreatAsAtomicUnit=on
  SlowFilTSeln_Mult12Temp : Subsystem  RequirementInfo={'linktype_rmi_doors' '0000a52a (/E-STEER Core/SubSystem Specifications/Application Functions/SF009A Thermal Duty Cycle Protection)' '#SF009A_151' 'true' 'REQ: SF009A_151' '' } %GIDa_a6dc9a2e_a1d7_4331_9833_20d4c5c34ffd  TreatAsAtomicUnit=on
  SlowFilTSeln_Mult36Temp : Subsystem  RequirementInfo={'linktype_rmi_doors' '0000a52a (/E-STEER Core/SubSystem Specifications/Application Functions/SF009A Thermal Duty Cycle Protection)' '#SF009A_151' 'true' 'REQ: SF009A_151' '' } %GIDa_6f859979_59ae_4faa_a03f_d836f73dc97e  TreatAsAtomicUnit=on
  StallCondition : Subsystem  RequirementInfo={'linktype_rmi_doors' '0000a52a (/E-STEER Core/SubSystem Specifications/Application Functions/SF009A Thermal Duty Cycle Protection)' '#SF009A_116' 'true' 'REQ: SF009A_116' '' } %GIDa_1316cb19_780c_427c_a230_3bcb89e7d51b  TreatAsAtomicUnit=on
  Mult1 : Outport  RequirementInfo={'linktype_rmi_doors' '0000a52a (/E-STEER Core/SubSystem Specifications/Application Functions/SF009A Thermal Duty Cycle Protection)' '#SF009A_155' 'true' 'REQ: SF009A_155' '' } %GIDa_fd8e61be_9bf0_4e18_a5e1_a43974329e69
  Mult2 : Outport  RequirementInfo={'linktype_rmi_doors' '0000a52a (/E-STEER Core/SubSystem Specifications/Application Functions/SF009A Thermal Duty Cycle Protection)' '#SF009A_155' 'true' 'REQ: SF009A_155' '' } %GIDa_35190f10_f645_47f4_8361_57d755b725f3  Port=2
  Mult3 : Outport  RequirementInfo={'linktype_rmi_doors' '0000a52a (/E-STEER Core/SubSystem Specifications/Application Functions/SF009A Thermal Duty Cycle Protection)' '#SF009A_155' 'true' 'REQ: SF009A_155' '' } %GIDa_c8fcc0c1_53bc_45d5_af25_a2bfad1812a3  Port=3
  Mult4 : Outport  RequirementInfo={'linktype_rmi_doors' '0000a52a (/E-STEER Core/SubSystem Specifications/Application Functions/SF009A Thermal Duty Cycle Protection)' '#SF009A_155' 'true' 'REQ: SF009A_155' '' } %GIDa_954126f0_9343_400e_8331_66461f78390e  Port=4
  Mult5 : Outport  RequirementInfo={'linktype_rmi_doors' '0000a52a (/E-STEER Core/SubSystem Specifications/Application Functions/SF009A Thermal Duty Cycle Protection)' '#SF009A_155' 'true' 'REQ: SF009A_155' '' } %GIDa_0c99cbdb_3a79_455c_847b_f10e0bf0b04c  Port=5
  Mult6 : Outport  RequirementInfo={'linktype_rmi_doors' '0000a52a (/E-STEER Core/SubSystem Specifications/Application Functions/SF009A Thermal Duty Cycle Protection)' '#SF009A_155' 'true' 'REQ: SF009A_155' '' } %GIDa_13beb251_3ba5_4222_af48_e6cae6175380  Port=6
  wires:
  Mult36Temp/1 -> SlowFilTSeln_Mult36Temp/1(Mult36Temp)
  Const1/1 -> If1/1
  MotVelCrf/1 -> Abslt_f32_f32/1
  Const2/1 -> If/2
  [Mult36TempSlc] -> NonStallCondition/2(Mult36TempSlc)
  Merge/1 -> Demux/1
  Demux/1 -> Data Store Write/1, Mult1/1  "Mult1"
  Demux/2 -> Data Store Write1/1, Mult2/1  "Mult2"
  Demux/3 -> Data Store Write2/1, Mult3/1  "Mult3"
  Demux/4 -> Data Store Write3/1, Mult4/1  "Mult4"
  Demux/5 -> Data Store Write4/1, Mult5/1  "Mult5"
  Demux/6 -> Data Store Write5/1, Mult6/1  "Mult6"
  Mult12Temp/1 -> [Mult12], SlowFilTSeln_Mult12Temp/1(Mult12Temp)
  [Mult12] -> NonStallCondition/1(Mult12Temp)
  Abslt_f32_f32/1 -> If/1
  [Mult36TempSlc] -> StallCondition/2(Mult36TempSlc)
  [Mult12] -> StallCondition/1(Mult12Temp)
  SlowFilTSeln_Mult12Temp/1(Mult36TempSlc) -> Merge1/1
  SlowFilTSeln_Mult36Temp/1(Mult36TempSlc) -> Merge1/2
  Merge1/1 -> [Mult36TempSlc]
  If1/1 -> SlowFilTSeln_Mult12Temp/Action
  If1/2 -> SlowFilTSeln_Mult36Temp/Action
  If/1 -> NonStallCondition/Action
  If/2 -> StallCondition/Action
  NonStallCondition/1(Mult) -> Merge/1
  StallCondition/1(Mult) -> Merge/2

== system SF009A_DutyCycThermProtn/DutyCycThermProtn/DutyCycThermProtnPer1/LoadLimiting/PowerOffTasks ==
  note: At power OFF, update NVM.
  CopyRight2 : Subsystem  Description=|  mask(Copyright Information){none=on}
      | Copyright info block.                                               
      |                                                                     
      | Place copyright information at the top of every subsystem in design.
      mask prompts: none "No parameters"
      mask help: Place copyright information at the top of every subsystem in design.
      mask Display:
      | NxtrConf = 'Nexteer Confidential';
      | 
      | sys = bdroot; %handle for the current model ("system")
      | first = get_param(sys,'Created');
      | first = first(end-3:end);  %year is last four digits
      | 
      | last = get_param(sys,'LastModifiedDate');
      | if isempty(last)
      |     last = datestr(now,'yyyy');
      | else
      |     last = last(end-3:end);
      | end
      | 
      | if strcmp(first,last)
      |     fprintf('%s -- Copyright %s Nexteer',NxtrConf,first)
      | else
      |     fprintf('%s -- %s%s- %s Nexteer',NxtrConf,char(169),first,last)
      | end
  Data Store Read1 : DataStoreRead  DataStoreName=Fild3Val  DataStoreElements=Fild3Val.FilSt
  Data Store Read2 : DataStoreRead  DataStoreName=Fild4Val  DataStoreElements=Fild4Val.FilSt
  Data Store Read3 : DataStoreRead  DataStoreName=Fild5Val  DataStoreElements=Fild5Val.FilSt
  Data Store Read4 : DataStoreRead  DataStoreName=Fild6Val  DataStoreElements=Fild6Val.FilSt
  Data Store Write : DataStoreWrite  DataStoreName=FilStVal  DataStoreElements=FilStVal.Fil3StVal
  Data Store Write1 : DataStoreWrite  DataStoreName=FilStVal  DataStoreElements=FilStVal.Fil4StVal
  Data Store Write2 : DataStoreWrite  DataStoreName=FilStVal  DataStoreElements=FilStVal.Fil5StVal
  Data Store Write3 : DataStoreWrite  DataStoreName=FilStVal  DataStoreElements=FilStVal.Fil6StVal
  Data Type Conversion{,1..3} (4 alike) : DataTypeConversion  OutDataTypeStr=uint8
  LimStat_f1 : NxtrLim/LimStat_f32  LoLim=FILVALMIN_ULS_F32  HiLim=FILVALMAX_ULS_F32
      settings: AttributesFormatString=Lower Limit: %<LoLim>\nUpper Limit: %<HiLim>
  LimStat_f2 : NxtrLim/LimStat_f32  LoLim=FILVALMIN_ULS_F32  HiLim=FILVALMAX_ULS_F32
      settings: AttributesFormatString=Lower Limit: %<LoLim>\nUpper Limit: %<HiLim>
  LimStat_f3 : NxtrLim/LimStat_f32  LoLim=FILVALMIN_ULS_F32  HiLim=FILVALMAX_ULS_F32
      settings: AttributesFormatString=Lower Limit: %<LoLim>\nUpper Limit: %<HiLim>
  LimStat_f32 : NxtrLim/LimStat_f32  RequirementInfo={} %GIDa_9cfebb92_a3ed_4173_aa17_612219a1860a  LoLim=FILVALMIN_ULS_F32  HiLim=FILVALMAX_ULS_F32
      settings: AttributesFormatString=Lower Limit: %<LoLim>\nUpper Limit: %<HiLim>
  wires:
  Data Store Read1/1 -> LimStat_f32/1
  LimStat_f32/1 -> Data Type Conversion/1
  LimStat_f1/1 -> Data Type Conversion1/1
  LimStat_f2/1 -> Data Type Conversion2/1
  LimStat_f3/1 -> Data Type Conversion3/1
  Data Store Read2/1 -> LimStat_f1/1
  Data Store Read3/1 -> LimStat_f2/1
  Data Store Read4/1 -> LimStat_f3/1
  Data Type Conversion/1 -> Data Store Write/1
  Data Type Conversion1/1 -> Data Store Write1/1
  Data Type Conversion2/1 -> Data Store Write2/1
  Data Type Conversion3/1 -> Data Store Write3/1
